simulink model "IntroToLQR_model"  (R2023a)
settings: Solver=VariableStepAuto  StartTime=0.0  StopTime=t_final  RelTol=1e-3
values from neighbouring files (symbols this model uses):
  A = [0 1 ... (first row only)    [LQR_tutorial.m]
  B = [0 ... (first row only)    [LQR_tutorial.m]
  x0 = [pi ... (first row only)    [LQR_tutorial.m]
undefined symbols (not defined in the file or in its folder): K
settings Model: Creator=Personal  LastModifiedBy=Personal

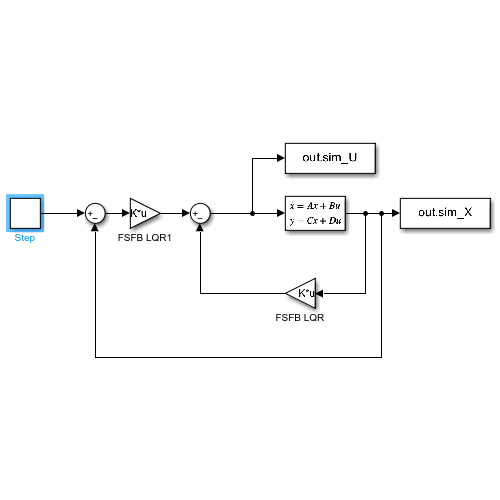
[thumbnail: Simulink's stored preview of the top-level diagram]
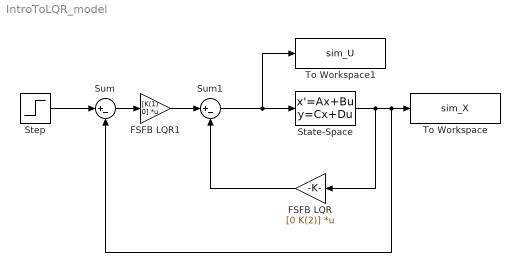
== system IntroToLQR_model ==
  FSFB LQR : Gain  Gain=[0 K(2)]  Multiplication=Matrix(K*u)
  FSFB LQR1 : Gain  Gain=[K(1) 0]  Multiplication=Matrix(K*u)
  State-Space : StateSpace  A=A  B=B  C=eye(2)  D=zeros(2,1)  InitialCondition=x0
  Step : Step  Time=0  After=2  SampleTime=0
  Sum : Sum  Inputs=|+-
  Sum1 : Sum  Inputs=|+-
  To Workspace : ToWorkspace  VariableName=sim_X  SaveFormat=Structure With Time  SampleTime=-1
  To Workspace1 : ToWorkspace  VariableName=sim_U  SaveFormat=Structure With Time  SampleTime=-1
  wires:
  State-Space/1 -> FSFB LQR/1, To Workspace/1, Sum/2
  FSFB LQR/1 -> Sum1/2
  Sum1/1 -> To Workspace1/1, State-Space/1
  Sum/1 -> FSFB LQR1/1
  Step/1 -> Sum/1
  FSFB LQR1/1 -> Sum1/1
